simulink model "idontKnow"  (R2018b)
settings: Solver=VariableStepAuto  StartTime=0.0  StopTime=500  MaxStep=1e-2  RelTol=1e-3
values from neighbouring files (symbols this model uses):
  A = [0,1;0,0]    [AAAA_trying.m]    (also in MPCController.m = plant.A; MPCController1.m; aaass.m; app1.m = 1)
  b = [0;1]    [AAAA_trying.m]    (also in aaass.m)
  B = plant.B    [MPCController.m]    (also in MPCController1.m = [0,0;1,-1]; aaass.m = [b,-b])
  C = plant.C    [MPCController.m]    (also in MPCController1.m = eye(2); aaass.m = eye(2))
  D = zeros(2,2)    [MPCController1.m]    (also in aaass.m)
  kd = 0.7021    [aaass.m]
  kp = 0.1859    [aaass.m]
  V = 1./(cT*inv(eye*(2) - Ad+bd*kT)*bd)    [aaass.m]
undefined symbols (not defined in the file or in its folder): K, loserloser, MPCController1
libraries: simulink x1
settings Model: Creator=HP  LastModifiedBy=HP

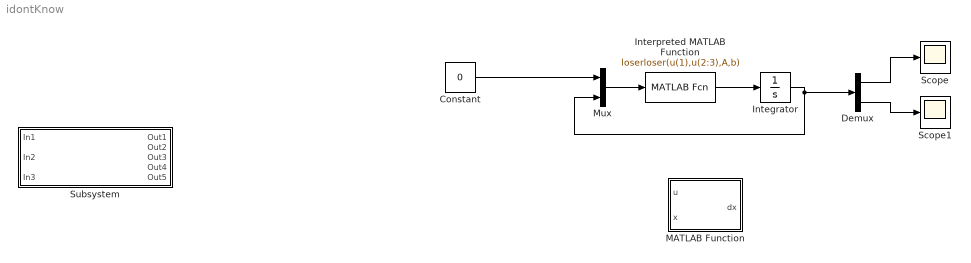
== system idontKnow ==
  Constant : Constant  Value=0
  Demux : Demux  Outputs=2
  Integrator : Integrator  InitialCondition=[0;20]
  Interpreted MATLAB Function : MATLABFcn  MATLABFcn=loserloser(u(1),u(2:3),A,b)
  MATLAB Function : MATLAB Function  TreatAsAtomicUnit=on
  Mux : Mux  Inputs=2
  Scope : Scope
  Scope1 : Scope
  Subsystem : Subsystem
  wires:
  Mux/1 -> Interpreted MATLAB Function/1
  Interpreted MATLAB Function/1 -> Integrator/1
  Constant/1 -> Mux/1
  Integrator/1 -> Mux/2, Demux/1
  Demux/1 -> Scope/1
  Demux/2 -> Scope1/1

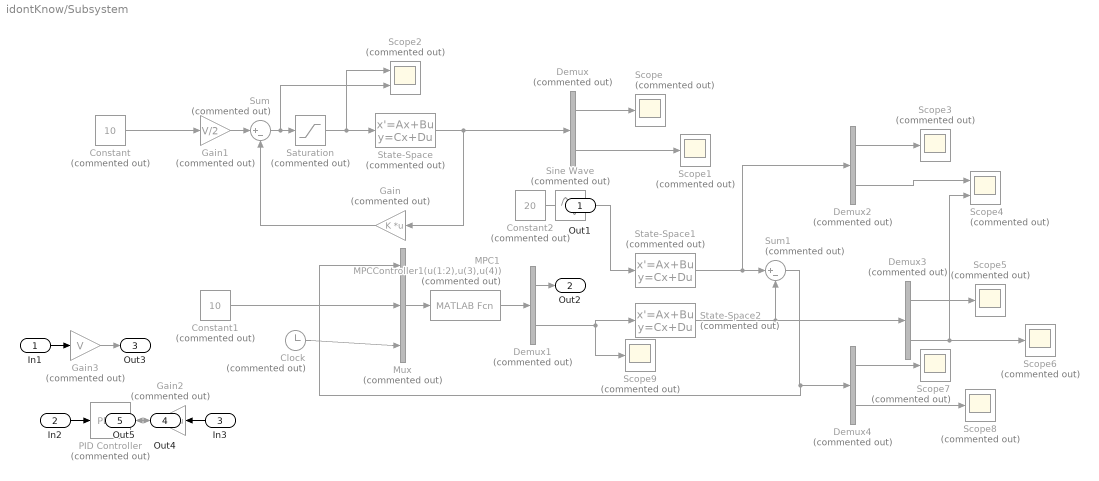
== system idontKnow/Subsystem ==
  In1 : Inport
  In2 : Inport  Port=2
  In3 : Inport  Port=3
  Clock : Clock  Commented=on
  Constant : Constant  Commented=on  Value=10
  Constant1 : Constant  Commented=on  Value=10
  Constant2 : Constant  Commented=on  Value=20
  Demux{,1..4} (5 alike) : Demux  Commented=on  Outputs=2
  Gain : Gain  Commented=on  Gain=K  Multiplication=Matrix(K*u)
  Gain1 : Gain  Commented=on  Gain=V/2
  Gain2 : Gain  Commented=on  Gain=K  Multiplication=Matrix(K*u)
  Gain3 : Gain  Commented=on  Gain=V
  MPC1 : MATLABFcn  Commented=on  MATLABFcn=MPCController1(u(1:2),u(3),u(4))  OutputDimensions=2
  Mux : Mux  Commented=on  Inputs=3
  PID Controller : simulink/Continuous/PID Controller  Commented=on  Controller=PD  Form=Parallel  TimeDomain=Continuous-time  SampleTime=-1  IntegratorMethod=Forward Euler  FilterMethod=Forward Euler  ControllerParametersSource=internal  P=-kp  I=1  D=-kd  UseFilter=on  N=100  TunerSelectOption=Transfer Function Based (PID Tuner App)  InitialConditionSource=internal  InitialConditionForIntegrator=0  InitialConditionForFilter=0  DifferentiatorICPrevScaledInput=0  ExternalReset=none  TrackingMode=off  Kt=1  LimitOutput=off  UpperSaturationLimit=inf  LowerSaturationLimit=-inf  LinearizeAsGain=on  AntiWindupMode=none  Kb=1  POutMin=[]  POutMax=[]  IOutMin=[]  IOutMax=[]  DOutMin=[]  DOutMax=[]  NOutMin=[]  NOutMax=[]  SumOutMin=[]  SumOutMax=[]  SaturationOutMin=[]  SaturationOutMax=[]  PParamMin=[]  PParamMax=[]  IParamMin=[]  IParamMax=[]  DParamMin=[]  DParamMax=[]  NParamMin=[]  NParamMax=[]  KbParamMin=[]  KbParamMax=[]  KtParamMin=[]  KtParamMax=[]  KbOutMin=[]  KbOutMax=[]  KtOutMin=[]  KtOutMax=[]  IntegratorOutMin=[]  IntegratorOutMax=[]  FilterOutMin=[]  FilterOutMax=[]  SumI1OutMin=[]  SumI1OutMax=[]  SumI2OutMin=[]  SumI2OutMax=[]  SumI3OutMin=[]  SumI3OutMax=[]  SumI4OutMin=[]  SumI4OutMax=[]  SumDOutMin=[]  SumDOutMax=[]  DifferentiatorOutMin=[]  DifferentiatorOutMax=[]  FilterDiffOutCoefMin=[]  FilterDiffOutCoefMax=[]  ReciprocalOutMin=[]  ReciprocalOutMax=[]  SumDenOutMin=[]  SumDenOutMax=[]  SumNumOutMin=[]  SumNumOutMax=[]  DivideOutMin=[]  DivideOutMax=[]  IntegratorContinuousStateAttributes=''  IntegratorStateMustResolveToSignalObject=off  IntegratorRTWStateStorageClass=Auto  FilterContinuousStateAttributes=''  FilterStateMustResolveToSignalObject=off  FilterRTWStateStorageClass=Auto  ParallelPVariant=InternalParameters  IdealPVariant=Disabled  IVariant=Disabled  DVariant=InternalParameters  IntegratorVariant=Disabled  SatVariant=Disabled  AWVariant=Disabled  PCopyVariant=Disabled  TRVariant=Disabled  FdbkBlocksVariant=Forward  IdealPFdbkVariant=Disabled  SatFdbkVariant=Disabled  DerivativeFilterVariant=ContFilter  NVariant=InternalParameters  NCopyVariant=Disabled  FilterICVariant=InternalICsFilter  IntegratorICVariant=Disabled  ExternalResetVariant=Disabled  TRSumVariant=Passthrough  SumFdbkVariant=Disabled  SumVariant=Sum_PD
  Saturation : Saturate  Commented=on  UpperLimit=5  LowerLimit=-8
  Scope{,1,3,5..9} (8 alike) : Scope  Commented=on
  Scope2 : Scope  Commented=on  NumInputPorts=2
  Scope4 : Scope  Commented=on  NumInputPorts=2
  Sine Wave : Sin  Commented=on  SampleTime=0
  State-Space : StateSpace  Commented=on  A=A  B=B  C=C  D=D  InitialCondition=[-50;-2]
  State-Space1 : StateSpace  Commented=on  A=A  B=b  C=eye(2)  D=zeros(2,1)  InitialCondition=[0;20]
  State-Space2 : StateSpace  Commented=on  A=A  B=b  C=eye(2)  D=zeros(2,1)  InitialCondition=[-100;20]
  Sum : Sum  Commented=on  Inputs=|+-
  Sum1 : Sum  Commented=on  Inputs=|+-
  Out1 : Outport
  Out2 : Outport  Port=2
  Out3 : Outport  Port=3
  Out4 : Outport  Port=4
  Out5 : Outport  Port=5
  wires:
  State-Space/1 -> Demux/1, Gain/1
  Demux1/2 -> State-Space2/1, Scope9/1
  State-Space2/1 -> Demux3/1, Sum1/2
  Demux/2 -> Scope1/1
  Constant/1 -> Gain1/1
  State-Space1/1 -> Demux2/1, Sum1/1
  Gain/1 -> Sum/2
  Demux/1 -> Scope/1
  Constant2/1 -> Out1/1
  Mux/1 -> MPC1/1
  Demux2/2 -> Scope4/1
  Demux3/1 -> Scope5/1
  Demux3/2 -> Scope4/2, Scope6/1
  Sum1/1 -> Mux/1, Demux4/1
  MPC1/1 -> Demux1/1
  Sum/1 -> Scope2/2, Saturation/1
  Gain1/1 -> Sum/1
  Demux1/1 -> Out2/1
  Saturation/1 -> Scope2/1, State-Space/1
  Demux4/1 -> Scope7/1
  Sine Wave/1 -> State-Space1/1
  Constant1/1 -> Mux/2
  PID Controller/1 -> Out4/1
  Gain3/1 -> Out3/1
  Demux4/2 -> Scope8/1
  Demux2/1 -> Scope3/1
  Clock/1 -> Mux/3
  In3/1 -> Gain2/1
  In2/1 -> PID Controller/1
  Gain2/1 -> Out5/1
  In1/1 -> Gain3/1

== matlab function idontKnow/MATLAB Function ==
  data: u input; dx output; x input; b parameter; A parameter
function dx = fcn(u,x,b, A)

dx = A*x + b*u;
